simulink model "SinglePhaseFullfBridge_inverter_RL"  (R2024b)
settings: Solver=FixedStepDiscrete  StartTime=0.0  StopTime=.1  FixedStep=Ts  RelTol=1e-3
InitFcn:
  | Ts=1e-5
  | f=50
libraries: spsIGBTDiodeLib x4, spsMeanLib x3, eeRmsMeasurement x2, spsSeriesRLCBranchLib x2, spsRMSLib x2, spsTHDLib x2, spsMultimeterLib x1, eePwmGenerator x1, spsSVPWMGenerator2LevelLib x1, spsSVPWMGenerator3LevelLib x1, spsDCVoltageSourceLib x1, spspowerguiLib x1
settings Model: Creator=ASINGH2  LastModifiedBy=diogo
settings SolverCC: AlgebraicLoopSolver=TrustRegion
settings DataIOCC: ReturnWorkspaceOutputs=off
settings OptimizationCC: ReuseModelBlockBuffer=off  LifeSpan=inf
settings DebuggingCC: SFExecutionAtInitializationDiag=none  ArithmeticOperatorsInVariantConditions=warning
settings ModelReferenceCC: EnableRefExpFcnMdlSchedulingChecks=on
settings SFSimCC: CustomCodeUndefinedFunction=UseInterfaceOnly
settings RTWCC: GPUComputeCapability=3.5  DLArmComputeVersion=19.05
settings CodeAppCC: StateflowObjectComments=on

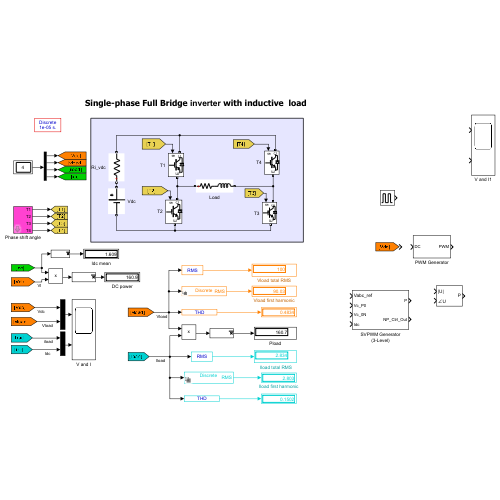
[thumbnail: Simulink's stored preview of the top-level diagram]
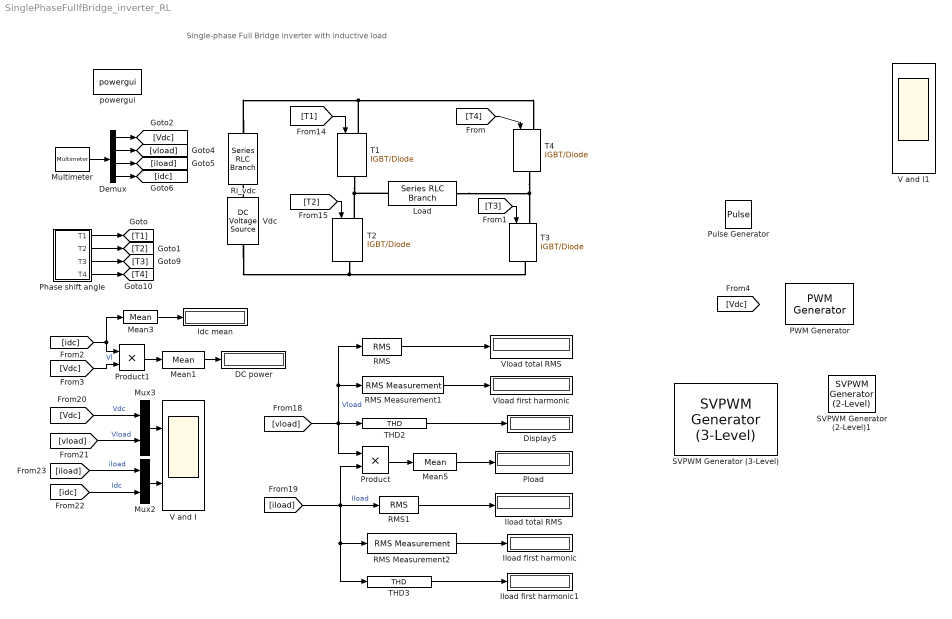
== system SinglePhaseFullfBridge_inverter_RL ==
  note: Single-phase Full Bridge inverter with inductive load
  " Iload total RMS" : Display
  " RMS Measurement2" : eeRmsMeasurement/RMS Measurement  LabelModeActiveChoice=Harmonic  F=f  SpecifyHarmonics=on  K=[1]  Ts=Ts
  DC power : Display
  Demux : Demux
  Display5 : Display
  Idc mean : Display
  Iload first harmonic : Display
  Iload first harmonic1 : Display
  Load : spsSeriesRLCBranchLib/Series RLC Branch  LConnTagsString=__new0  RConnTagsString=__new0  BranchType=RL  Resistance=20  Inductance=8e-2  SetiL0=off  InitialCurrent=0  Capacitance=1e-6  Setx0=off  InitialVoltage=0  Measurements=Branch voltage and current
  Mean1 : spsMeanLib/Mean  Freq=f  Vinit=0  Ts=Ts
  Mean3 : spsMeanLib/Mean  Freq=f  Vinit=0  Ts=Ts
  Mean5 : spsMeanLib/Mean  Freq=f  Vinit=0  Ts=Ts
  Multimeter : spsMultimeterLib/Multimeter  L=4  sel=[2 1 3 4]  yselected={}  Gain=[1 1 1 1]  OutputType=Complex  PlotAtSimulationStop=off  PhasorSimulation=off
  Mux2 : Mux  Inputs=2
  Mux3 : Mux  Inputs=2
  PWM Generator : eePwmGenerator/PWM Generator  CarrCount=Up  Tper=0.001  Tdelay=0  Ts=Ts
  Phase shift angle : Subsystem  mask{teta=0}
      mask prompts: teta "Phase Shift angle (in degrees)"
  Pload : Display
  Product : Product
  Product1 : Product
  Pulse Generator : DiscretePulseGenerator  PulseType=Time based  Period=10  PulseWidth=5
  RMS : spsRMSLib/RMS  TrueRMS=on  Freq=f  RMSInit=0  Ts=Ts
  RMS Measurement1 : eeRmsMeasurement/RMS Measurement  LabelModeActiveChoice=Harmonic  F=f  SpecifyHarmonics=on  K=[1]  Ts=Ts
  RMS1 : spsRMSLib/RMS  TrueRMS=on  Freq=f  RMSInit=0  Ts=Ts
  Ri_vdc : spsSeriesRLCBranchLib/Series RLC Branch  LConnTagsString=__new0  RConnTagsString=__new0  BranchType=R  Resistance=0.0000001  Inductance=1e-3  SetiL0=off  InitialCurrent=0  Capacitance=1e-6  Setx0=off  InitialVoltage=0  Measurements=Branch current
  SVPWM Generator (2-Level)1 : spsSVPWMGenerator2LevelLib/SVPWM Generator (2-Level)  InputType=Magnitude-Angle (rad)  SwitchingPattern=Pattern #1  Fc=2000  ParUref=[0.8 -30 50]  Ts=0
  SVPWM Generator (3-Level) : spsSVPWMGenerator3LevelLib/SVPWM Generator (3-Level)  InputType=Three-phase signals  Kp=0.04  fn=30  Fsw=1620  ParVref=[0.8 -30 60]  Ts=0
      settings: LibrarySourceBlock=|
      | sps_lib/Power Electronics/Power Electronics Control/SVPWM Generator
      | (3-Level)
  T{1..4} (4 alike) : spsIGBTDiodeLib/IGBT//Diode  Ron=1e-6  Rs=1e5  Cs=inf  Measurements=off
  THD2 : spsTHDLib/THD  Freq=f  Ts=Ts
  THD3 : spsTHDLib/THD  Freq=f  Ts=Ts
  V and I : Scope  NumInputPorts=2
  V and I1 : Scope  NumInputPorts=2
  Vdc : spsDCVoltageSourceLib/DC Voltage Source  Amplitude=100  Measurements=Voltage
  Vload first harmonic : Display
  Vload total RMS : Display
  powergui : spspowerguiLib/powergui  Priority=1  SimulationMode=Discrete  SampleTime=Ts  frequency=60  Iterations=50  frequencyindice=0  Pbase=100e6  ErrMax=1e-4  UnitsV=kV  UnitsW=MW  buscounter=0  FunctionMessages=off  echomessages=off  EnableUseOfTLC=off  CurrentSourceSwitches=off  DisableSnubberDevices=off  DisableRonSwitches=off  DisableVfSwitches=off  DisplayEquations=off  AutomaticDiscreteSolvers=off  SolverType=Tustin/Backward Euler (TBE)  Interpol=off  ExternalGateDelay=off  methode=off  Ts=100  x0status=blocks  SPID=on  SwTol=0  HookPort=off  NonlinearTolerance=0  nMaxIteration=15  ContinueOnMaxIteration=off  RestoreLinks=warning  ResistiveCurrentMeasurement=off  Frange=[0:2:500]  Ylog=off  Xlog=on  ShowGrid=off  save=off  variable=ZData  structure=0  ZoomFFT=off  StartTime=0.0  cycles=1  DisplayStyle=1  fundamental=60  FreqAxis=off  MaxFrequency=1000  frequencyindicesteady=1  RmsSteady=1  display=off
  wires:
  Phase shift angle/1(T1) -> [T1]
  Phase shift angle/2(T2) -> [T2]
  [T4] -> T4/1
  [T3] -> T3/1
  Multimeter/1 -> Demux/1
  Demux/2 -> [vload]
  Demux/3 -> [iload]
  Demux/4 -> [idc]
  Phase shift angle/3(T3) -> [T3]
  Phase shift angle/4(T4) -> [T4]
  [T1] -> T1/1
  [T2] -> T2/1
  [iload] -> Mux2/1  "iload"
  [iload] -> Product/2, THD3/1, " RMS Measurement2"/1, RMS1/1  "Iload"
  RMS Measurement1/1 -> Vload first harmonic/1
  Mean5/1 -> Pload/1
  RMS1/1 -> " Iload total RMS"/1
  [vload] -> Product/1, RMS/1, RMS Measurement1/1, THD2/1  "Vload"
  Mux2/1 -> V and I/2
  Product/1 -> Mean5/1
  Mux3/1 -> V and I/1
  [Vdc] -> Mux3/1  "Vdc"
  [idc] -> Mux2/2  "Idc"
  [vload] -> Mux3/2  "Vload"
  Demux/1 -> [Vdc]
  RMS/1 -> Vload total RMS/1
  THD2/1 -> Display5/1
  Mean1/1 -> DC power/1
  [Vdc] -> Product1/2  "Vl"
  Product1/1 -> Mean1/1
  [idc] -> Mean3/1, Product1/1
  Mean3/1 -> Idc mean/1
  " RMS Measurement2"/1 -> Iload first harmonic/1
  THD3/1 -> Iload first harmonic1/1
  connections:
  T1/LConn1 -- Ri_vdc/RConn1 -- T4/LConn1
  T4/RConn1 -- Load/RConn1 -- T3/LConn1
  Load/LConn1 -- T2/LConn1 -- T1/RConn1
  Vdc/LConn1 -- T3/RConn1 -- T2/RConn1
  Vdc/RConn1 -- Ri_vdc/LConn1

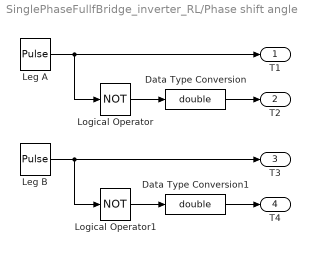
== system SinglePhaseFullfBridge_inverter_RL/Phase shift angle ==
  Data Type Conversion : DataTypeConversion  OutDataTypeStr=double  SaturateOnIntegerOverflow=off  RndMeth=Floor
  Data Type Conversion1 : DataTypeConversion  OutDataTypeStr=double  SaturateOnIntegerOverflow=off  RndMeth=Floor
  Leg A : DiscretePulseGenerator  Period=round(1/f/Ts)  PulseWidth=round(1/f/Ts/2)  SampleTime=Ts
  Leg B : DiscretePulseGenerator  Period=round(1/f/Ts)  PulseWidth=round(1/f/Ts/2)  PhaseDelay=round(1000*teta/180)  SampleTime=Ts
  Logical Operator : Logic  Operator=NOT  IconShape=distinctive  AllPortsSameDT=off  OutDataTypeStr=boolean
  Logical Operator1 : Logic  Operator=NOT  IconShape=distinctive  AllPortsSameDT=off  OutDataTypeStr=boolean
  T1 : Outport  VectorParamsAs1DForOutWhenUnconnected=off
  T2 : Outport  Port=2  VectorParamsAs1DForOutWhenUnconnected=off
  T3 : Outport  Port=3  VectorParamsAs1DForOutWhenUnconnected=off
  T4 : Outport  Port=4  VectorParamsAs1DForOutWhenUnconnected=off
  wires:
  Leg A/1 -> T1/1, Logical Operator/1
  Logical Operator/1 -> Data Type Conversion/1
  Data Type Conversion/1 -> T2/1
  Data Type Conversion1/1 -> T4/1
  Logical Operator1/1 -> Data Type Conversion1/1
  Leg B/1 -> Logical Operator1/1, T3/1
